simulink model "Accelerator"  (R2022b)
settings: Solver=FixedStepDiscrete  StartTime=0.0  StopTime=10  FixedStep=0.005  RelTol=1e-3  EnableMultiTasking=on
PreLoadFcn:
  | try, model_open; catch, disp('Error occurred while executing model pre-load callback: model_open.m'); disp('Please assure that the MATLAB working directory is set to the model directory before opening.'); end
InitFcn:
  | try, model_open; catch, end
undefined symbols (not defined in the file): GCM, raptor_get_safe_string, raptor_xcp_function
libraries: Raptor_lib x149, simulink x14, Blocks_Library x2, simulink_extras x1
(part 2 of 3)

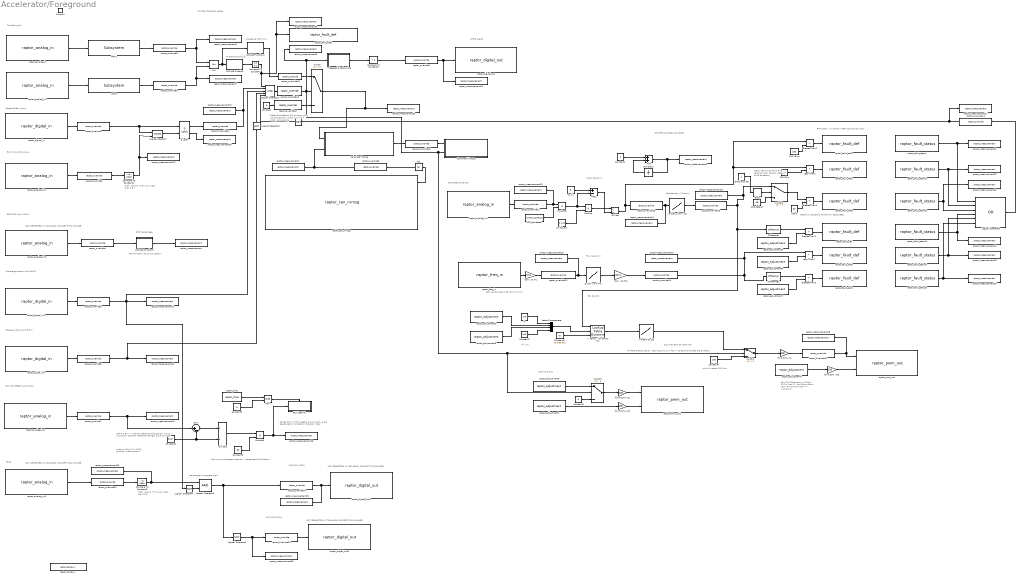
== system Accelerator/Foreground ==
  note: Pre-charge in progress logic
  note: IMD OKHS COIL-
  note: TSMS
  note: NOT REFLECTED IN TOP-LEVEL: COMPETITION CHANGE
  note: Fault function (for some reason)
  note: Throttle enable signal - cooling turns on when Inverter and throttle are enabled
  note: Cooling Pump
  note: Can handle about 4Hz at minimum
  note: Delay temp high fault for 5 seconds upon startup, default to 25 at startup
  note: Resistance in kilo-ohm
  note: Range from +/-50A
      | Negative and positive are dependent on direction of sensor install
  note: Defaults throttle to 0% on error, do not change this unless you know what you're doing
  note: Maximum amperage of sensor, independent of direction
  note: Linearity Error = +/-0.5%
      | Ignored in calculations
  note: Vref = 2.5V --> internal reference
      | Change this value if using an external reference:
      | Range is 0.5 to 2.65V
  note: Averaging POT1 & 2
  note: Throttle Plausibility
  note: Temperature Sensor
  note: Throttle Input
  note: SYSTEM CONTROL CODE
  note: SOC Percentage
  note: High: Above ~2.5V
      | Low: Less than 2.5V
  note: Starter Button Input
  note: Error Input
      | Active Low
  note: BMS SOC Input
      | (0-5V)
  note: Pre-charge Status input
      | (0-5V)
  note: Charge mode input
      | (0-5V)
  note: RTDS Signal
  note: Hold inverted PWM low
  note: Based on Cascadia and Emrax datasheets
  note: Persistent - will remain after VCU power cycle
  note: All in F
  note: assumes 80W @ 100% DC
  note: Flow Sensor In
  note: Fan PWM Frequency is 24KHz
      | 5/(2*pi*tau) --> tau=Larm/Rarm
      | Larm = 0.137mH
      | Rarm = 4.114ohm
  note: Temp Sensor In
  note: Fan Control
  note: DRIVETRAIN COOLING CODE
  note: GLV Hall Effect Input
      | (0-5V)
  note: NOT REFLECTED IN TOP-LEVEL: COMPETITION CHANGE
  note: NOT REFLECTED IN TOP-LEVEL: COMPETITION CHANGE
  note: NOT REFLECTED IN TOP-LEVEL: COMPETITION CHANGE
  note: IMD GLV+ COIL-
  note: High: Above ~2.2V
      | Low: Less than 2.2V
  function : TriggerPort  TriggerType=function-call  VariantControl=(inherit)
  100 C : Constant  Value=80
  100 Ohm : Constant  Value=0.1
  100 kOhm : Constant  Value=100
  25C default : Constant  Value=25
  ADC_corrected : Constant  Value=0.00122100122
  Abs : Abs  SaturateOnIntegerOverflow=off
  Add : Sum
  Add2 : Sum  Inputs=+-
  Calculate Torque : Subsystem
  Command Troque : Subsystem
  Compare To Constant : simulink/Logic and Bit Operations/Compare To Constant  relop=<=  const=0.1  OutDataTypeStr=boolean
  Compare To Constant1 : simulink/Logic and Bit Operations/Compare To Constant  relop=>=  const=2000  OutDataTypeStr=boolean
  Compare To Constant2 : simulink/Logic and Bit Operations/Compare To Constant  relop=>  const=0  OutDataTypeStr=boolean
  Compare To Constant3 : simulink/Logic and Bit Operations/Compare To Constant  relop=>=  const=1800  OutDataTypeStr=boolean
  Constant : Constant  Value=0
  Constant1 : Constant
  Constant2 : Constant  Value=2047
  Constant3 : Constant  Value=50
  Constant4 : Constant  Value=100
  Constant5 : Constant  Value=[0;0;80;80]
  Constant6 : Constant  Value=0
  Constant7 : Constant  Value=149
  Constant8 : Constant  Value=.5
  Conv. to Hz : Gain  Gain=0.01  OutDataTypeStr=uint32  RndMeth=Nearest
  Conv. to Hz1 : Gain  Gain=227.1  OutDataTypeStr=uint32
  D Latch : simulink_extras/Flip Flops/D Latch
  Delay : Delay  DelayLength=1000  InitialCondition=0
  Difference : simulink/Discrete/Difference  ICPrevInput=0.0  OutMin=[]  OutMax=[]  OutDataType=fixdt(1, 16)  OutScaling=2^-10  DoSatur=off
  Difference1 : simulink/Discrete/Difference  ICPrevInput=0.0  OutMin=[]  OutMax=[]  OutDataType=fixdt(1, 16)  OutScaling=2^-10  DoSatur=off
  Divide : Product  Inputs=*/
  Divide1 : Product  Inputs=*/
  Enable switch : Constant
  F : Constant  Value=-18
  GLV Used Ah : Subsystem  TreatAsAtomicUnit=on
  GreaterThan{1..4} (4 alike) : RelationalOperator  Operator=>  OutDataTypeStr=boolean  RndMeth=Simplest  InputSameDT=off
  I: 0-80W O: DC : Lookup_n-D  NumberOfTableDimensions=1  BreakpointsForDimension1=[0;5;10;15;20;25;30;35;40;45;50;55;60;65;70;75;80]  Table=[100;93.75;87.5;81.25;75;68.75;62.5;56.25;50;43.75;37.5;31.25;25;18.75;12.5;6.25;0]  InternalRulePriority=Speed  RndMeth=Simplest
  I: R (kOhm) O: T (C) : Lookup_n-D  NumberOfTableDimensions=1  BreakpointsForDimension1=[0.583;0.6601;0.7487;0.8508;0.9688;1.106;1.265;1.452;1.67;1.928;2.232;2.593;3.025;3.541;4.163;4.914;5.827;6.942;8.311;10;12.1;14.71;17.99;22.13;27.39]  Table=[120;115;110;105;100;95;90;85;80;75;70;65;60;55;50;45;40;35;30;25;20;15;10;5;0]  InternalRulePriority=Speed  RndMeth=Simplest
  I: Temp. () O: Power (W) : simulink/Lookup Tables/Lookup Table Dynamic  LookUpMeth=Interpolation-Use End Values  OutDataType=fixdt('double')  OutScaling=[]  OutputDataTypeScalingMode=Specify via dialog  OutDataTypeStr=double  DoSatur=off
  Less Than1 : RelationalOperator  Operator=<  OutDataTypeStr=boolean  RndMeth=Simplest  InputSameDT=off
  Less Than2 : RelationalOperator  Operator=<  OutDataTypeStr=boolean  RndMeth=Simplest  InputSameDT=off
  Logical Operator : Logic  Operator=NXOR  IconShape=distinctive  AllPortsSameDT=off  OutDataTypeStr=boolean
  Logical Operator1 : Logic  Inputs=5  IconShape=distinctive  AllPortsSameDT=off  OutDataTypeStr=boolean
  Logical Operator{2,4,6..7} (4 alike) : Logic  Operator=NOT  IconShape=distinctive  AllPortsSameDT=off  OutDataTypeStr=boolean
  Logical Operator3 : Logic  Operator=OR  Inputs=6  IconShape=distinctive  AllPortsSameDT=off  OutDataTypeStr=boolean
  Logical Operator5 : Logic  IconShape=distinctive  AllPortsSameDT=off  OutDataTypeStr=boolean
  MATLAB Function : MATLAB Function  TreatAsAtomicUnit=on
  MATLAB Function1 : MATLAB Function  TreatAsAtomicUnit=on
  MATLAB Function2 : MATLAB Function  TreatAsAtomicUnit=on
  Mod : Math  Operator=mod  OutputSignalType=real
  Mux : Mux  Inputs=2
      settings: DisplayOption=signals
  POT1 : Blocks_Library/Subsystem  nam=POT1
  POT2 : Blocks_Library/Subsystem  nam=POT2
  PU (Ohms) : Constant  Value=2.145
  Product : Product
  Product1 : Product
  Product3 : Product
  Q (L/H) vs. F (Hz) : Lookup_n-D  NumberOfTableDimensions=1  BreakpointsForDimension1=[16;32.5;49.3;65.5;82;90.2]  Table=[120;240;360;480;600;720]  ExtrapMethod=Clip  InternalRulePriority=Speed  OutDataTypeStr=double  RndMeth=Simplest
  Sum : Sum  Inputs=|+-
  Switch : Switch  Threshold=1  SaturateOnIntegerOverflow=off  InputSameDT=off
  Switch1 : Switch  Criteria=u2 > Threshold  SaturateOnIntegerOverflow=off  InputSameDT=off
  Switch2 : Switch  Criteria=u2 > Threshold  SaturateOnIntegerOverflow=off  InputSameDT=off
  Switch3 : Switch  Criteria=u2 > Threshold  SaturateOnIntegerOverflow=off  InputSameDT=off
  Triggered Single Pulse : Subsystem  Description=Produce a signal pulse for the RTDS timer circuit  TreatAsAtomicUnit=on  mask(single pulse generation){p_wid=5}
      mask prompts: p_wid "pulse width (number of samples)"
      mask help: This block generate a single pulse whenever a trigger happen. The pulse width must specified as a number of samples. for example if your sampling time is 0.1s and you want 3s pulse , then you should enter 30 as a pulse width.
      mask Display:
      | plot([0],[0])
      | plot([11],[0])
      | plot([5],[0.5])
      | plot([4 5 5 6 6 7],[0 0 0.25 0.25 0 0])
      | plot([5],[-0.3])
      | 
      | port_label('output', 1, 'Pulse')
      | port_label('input', 1, 'Trigger')
  Unit Delay : UnitDelay  SampleTime=-1  HasFrameUpgradeWarning=on
  Vector Concatenate : Concatenate  NumInputs=4
  Vs (V) : Constant  Value=5
  for 0.01% inc{,1..3} (4 alike) : Gain  Gain=100  OutDataTypeStr=Inherit: Inherit via back propagation
  raptor_adjustment1 : Raptor_lib/Data Storage/raptor_adjustment  paramName='Pump_PWM_freq'  nameSource=Parameter  initValue=24000  dataType=uint32  storage=Calibration  calDispType=Number  calEnum={'False', 'True'}  calGain=100  calOffset=0.0  calMax=inf  calMin=-inf  calFormat='-1'  calUnit='Hz'  calHelp=''  calAccess=1  calFunction=raptor_xcp_function(gcb)  calDispHeaders=off  calColHeaders={'Col1' 'Col2' 'Col3'}  calRowHeaders={'Row1' 'Row2' 'Row3'}
      settings: SourceProductName=Raptor
  raptor_adjustment2 : Raptor_lib/Data Storage/raptor_adjustment  paramName='LowerFanPoint'  nameSource=Parameter  initValue=18  dataType=double  storage=Calibration  calDispType=Number  calEnum={'False', 'True'}  calGain=1.0  calOffset=0.0  calMax=inf  calMin=-inf  calFormat='-1'  calUnit='F'  calHelp='Temp at 0W'  calAccess=1  calFunction=raptor_xcp_function(gcb)  calDispHeaders=off  calColHeaders={'Col1' 'Col2' 'Col3'}  calRowHeaders={'Row1' 'Row2' 'Row3'}
      settings: SourceProductName=Raptor
  raptor_adjustment3 : Raptor_lib/Data Storage/raptor_adjustment  paramName='UpperFanPoint'  nameSource=Parameter  initValue=66  dataType=double  storage=Calibration  calDispType=Number  calEnum={'False', 'True'}  calGain=1.0  calOffset=0.0  calMax=inf  calMin=-inf  calFormat='-1'  calUnit='F'  calHelp='Temp at 80W'  calAccess=1  calFunction=raptor_xcp_function(gcb)  calDispHeaders=off  calColHeaders={'Col1' 'Col2' 'Col3'}  calRowHeaders={'Row1' 'Row2' 'Row3'}
      settings: SourceProductName=Raptor
  raptor_adjustment4 : Raptor_lib/Data Storage/raptor_adjustment  paramName='Fan_PWM_freq'  nameSource=Parameter  initValue=24000  dataType=uint32  storage=Calibration  calDispType=Number  calEnum={'False', 'True'}  calGain=100  calOffset=0.0  calMax=inf  calMin=-inf  calFormat='-1'  calUnit='Hz'  calHelp=''  calAccess=1  calFunction=raptor_xcp_function(gcb)  calDispHeaders=off  calColHeaders={'Col1' 'Col2' 'Col3'}  calRowHeaders={'Row1' 'Row2' 'Row3'}
      settings: SourceProductName=Raptor
  raptor_adjustment5 : Raptor_lib/Data Storage/raptor_adjustment  paramName='tempRateFault'  nameSource=Parameter  initValue=10  dataType=double  storage=Calibration  calDispType=Number  calEnum={'False', 'True'}  calGain=1.0  calOffset=0.0  calMax=inf  calMin=-inf  calFormat='-1'  calUnit='degC/sec'  calHelp=''  calAccess=1  calFunction=raptor_xcp_function(gcb)  calDispHeaders=off  calColHeaders={'Col1' 'Col2' 'Col3'}  calRowHeaders={'Row1' 'Row2' 'Row3'}
      settings: SourceProductName=Raptor
  raptor_adjustment6 : Raptor_lib/Data Storage/raptor_adjustment  paramName='lowFlowRateFault'  nameSource=Parameter  initValue=1  dataType=double  storage=Calibration  calDispType=Number  calEnum={'False', 'True'}  calGain=1.0  calOffset=0.0  calMax=inf  calMin=-inf  calFormat='-1'  calUnit='GPM'  calHelp=''  calAccess=1  calFunction=raptor_xcp_function(gcb)  calDispHeaders=off  calColHeaders={'Col1' 'Col2' 'Col3'}  calRowHeaders={'Row1' 'Row2' 'Row3'}
      settings: SourceProductName=Raptor
  raptor_adjustment7 : Raptor_lib/Data Storage/raptor_adjustment  paramName='eradicFlowRateFault'  nameSource=Parameter  initValue=10  dataType=double  storage=Calibration  calDispType=Number  calEnum={'False', 'True'}  calGain=1.0  calOffset=0.0  calMax=inf  calMin=-inf  calFormat='-1'  calUnit='deg/sec'  calHelp=''  calAccess=1  calFunction=raptor_xcp_function(gcb)  calDispHeaders=off  calColHeaders={'Col1' 'Col2' 'Col3'}  calRowHeaders={'Row1' 'Row2' 'Row3'}
      settings: SourceProductName=Raptor
  raptor_adjustment8 : Raptor_lib/Data Storage/raptor_adjustment  paramName='Cooling_pump_PWM_D'  nameSource=Parameter  initValue=0.4  dataType=double  storage=Calibration  calDispType=Number  calEnum={'False', 'True'}  calGain=1.0  calOffset=0.0  calMax=inf  calMin=-inf  calFormat='-1'  calUnit='F'  calHelp='Temp at 80W'  calAccess=1  calFunction=raptor_xcp_function(gcb)  calDispHeaders=off  calColHeaders={'Col1' 'Col2' 'Col3'}  calRowHeaders={'Row1' 'Row2' 'Row3'}
      settings: SourceProductName=Raptor
  raptor_analog_in : Raptor_lib/Input & Output/raptor_analog_in  resourceValues=INPUT2|INPUT3|INPUT4|INPUT5|INPUT6|INPUT7|INPUT8|INPUT9|INPUT10|INPUT11|INPUT12|INPUT13|INPUT14|INPUT15|INPUT16|INPUT17|INPUT18|INPUT19|INPUT20|INPUT21|INPUT22|INPUT23|INPUT24|INPUT25|INPUT26|INPUT27|INPUT28|INPUT29|INPUT30|INPUT31|INPUT32|(None)  resource=INPUT30  rangeValues=0 - 5 V  range=0 - 5 V  filterrateValues=[]  filterrate='RAPTOR MASK DEFAULT'  resolutionValues=[]  resolution=[]  pullUDValues=215k PD  pullUD=215k PD
      settings: SourceProductName=Raptor
  raptor_analog_in1 : Raptor_lib/Input & Output/raptor_analog_in  resourceValues=INPUT2|INPUT3|INPUT4|INPUT5|INPUT6|INPUT7|INPUT8|INPUT9|INPUT10|INPUT11|INPUT12|INPUT13|INPUT14|INPUT15|INPUT16|INPUT17|INPUT18|INPUT19|INPUT20|INPUT21|INPUT22|INPUT23|INPUT24|INPUT25|INPUT26|INPUT27|INPUT28|INPUT29|INPUT30|INPUT31|INPUT32|(None)  resource=INPUT29  rangeValues=0 - 5 V  range=0 - 5 V  filterrateValues=[]  filterrate='RAPTOR MASK DEFAULT'  resolutionValues=[]  resolution=[]  pullUDValues=215k PD  pullUD=215k PD
      settings: SourceProductName=Raptor
  raptor_analog_in2 : Raptor_lib/Input & Output/raptor_analog_in  resourceValues=INPUT2|INPUT3|INPUT4|INPUT5|INPUT6|INPUT7|INPUT8|INPUT9|INPUT10|INPUT11|INPUT12|INPUT13|INPUT14|INPUT15|INPUT16|INPUT17|INPUT18|INPUT19|INPUT20|INPUT21|INPUT22|INPUT23|INPUT24|INPUT25|INPUT26|INPUT27|INPUT28|INPUT29|INPUT30|INPUT31|INPUT32|(None)  resource=INPUT23  rangeValues=0 - 5 V  range=0 - 5 V  filterrateValues=[]  filterrate='RAPTOR MASK DEFAULT'  resolutionValues=[]  resolution=[]  pullUDValues=56.7k PD  pullUD=56.7k PD
      settings: SourceProductName=Raptor
  raptor_analog_in3 : Raptor_lib/Input & Output/raptor_analog_in  resourceValues=INPUT2|INPUT3|INPUT4|INPUT5|INPUT6|INPUT7|INPUT8|INPUT9|INPUT10|INPUT11|INPUT12|INPUT13|INPUT14|INPUT15|INPUT16|INPUT17|INPUT18|INPUT19|INPUT20|INPUT21|INPUT22|INPUT23|INPUT24|INPUT25|INPUT26|INPUT27|INPUT28|INPUT29|INPUT30|INPUT31|INPUT32|(None)  resource=INPUT25  rangeValues=0 - 5 V  range=0 - 5 V  filterrateValues=[]  filterrate='RAPTOR MASK DEFAULT'  resolutionValues=[]  resolution=[]  pullUDValues=2.15k PU  pullUD=2.15k PU
      settings: SourceProductName=Raptor
  raptor_analog_in4 : Raptor_lib/Input & Output/raptor_analog_in  resourceValues=INPUT2|INPUT3|INPUT4|INPUT5|INPUT6|INPUT7|INPUT8|INPUT9|INPUT10|INPUT11|INPUT12|INPUT13|INPUT14|INPUT15|INPUT16|INPUT17|INPUT18|INPUT19|INPUT20|INPUT21|INPUT22|INPUT23|INPUT24|INPUT25|INPUT26|INPUT27|INPUT28|INPUT29|INPUT30|INPUT31|INPUT32|(None)  resource=INPUT21  rangeValues=0 - 5 V  range=0 - 5 V  filterrateValues=[]  filterrate='RAPTOR MASK DEFAULT'  resolutionValues=[]  resolution=[]  pullUDValues=2.15k PU  pullUD=2.15k PU
      settings: SourceProductName=Raptor
  raptor_analog_in5 : Raptor_lib/Input & Output/raptor_analog_in  resourceValues=INPUT2|INPUT3|INPUT4|INPUT5|INPUT6|INPUT7|INPUT8|INPUT9|INPUT10|INPUT11|INPUT12|INPUT13|INPUT14|INPUT15|INPUT16|INPUT17|INPUT18|INPUT19|INPUT20|INPUT21|INPUT22|INPUT23|INPUT24|INPUT25|INPUT26|INPUT27|INPUT28|INPUT29|INPUT30|INPUT31|INPUT32|(None)  resource=INPUT26  rangeValues=0 - 5 V  range=0 - 5 V  filterrateValues=[]  filterrate='RAPTOR MASK DEFAULT'  resolutionValues=[]  resolution=[]  pullUDValues=681k PU  pullUD=681k PU
      settings: SourceProductName=Raptor
  raptor_analog_in6 : Raptor_lib/Input & Output/raptor_analog_in  resourceValues=INPUT2|INPUT3|INPUT4|INPUT5|INPUT6|INPUT7|INPUT8|INPUT9|INPUT10|INPUT11|INPUT12|INPUT13|INPUT14|INPUT15|INPUT16|INPUT17|INPUT18|INPUT19|INPUT20|INPUT21|INPUT22|INPUT23|INPUT24|INPUT25|INPUT26|INPUT27|INPUT28|INPUT29|INPUT30|INPUT31|INPUT32|(None)  resource=INPUT24  rangeValues=0 - 5 V  range=0 - 5 V  filterrateValues=[]  filterrate='RAPTOR MASK DEFAULT'  resolutionValues=[]  resolution=[]  pullUDValues=56.7k PD  pullUD=56.7k PD
      settings: SourceProductName=Raptor
  raptor_can_rxmsg : Raptor_lib/CAN/raptor_can_rxmsg  canDefinition=struct('dbcFile', '20210505 RMS PM and RM CAN DB.dbc','message', 'M165_Motor_Position_Info','comment', '','signals', {{'D1_Motor_Angle_Electrical','D2_Motor_Speed','D3_Electrical_Output_Frequency','D4_Delta_Resolver_Filtered'}},'enabled', [ 1 1 1 1;],'scaled', [ 1 1 1 1;],'canBus', '''CAN1''','messageID', [ 165;],'idMask', [ 536870911;],'payloadMask', [],'payloadValue', [],'period', [ 0;],'mailbox', '''''','queueSize', [ 1;],'label', [ 0;],'ver', [ 2;],'showID', [ 0;],'showRaw', [ 0;],'showRawMsg', [ 0;],'useStartVals', [ 0;],'extendedId', [ 0;],'showAge', [ 0;],'useSimFunc', [ 0;],'sim_func_name', '''''','fill', [ 0;],'editID', [ 0;],'signalOrder', [ 1;],'signalAscDes', [ 1;],'msgLength', [ 8;])  canBus='CAN1'  mailbox=''  payloadMask=[]  payloadValue=[]  idMask=hex2dec('1FFFFFFF')  queueSize=1  showID=0  label=0  fill=0  id=165  showRaw=0  showAge=0  signalOrder=1  signalInfo={{struct('Name', 'D4_Delta_Resolver_Filtered','StartBit', [ 48;],'SignalSize', [ 16;],'ByteOrder', 'LittleEndian','ValueType', 'SIGNED','Class', 'int16','Signed', [ 1;],'Factor', [ 0.1;],'Offset', [ 0;],'Min', [ -3276.8;],'Max', [ 3276.7;],'Units', 'deg','StartVal', [ 0;],'Comment', 'Used in calibration of resolver angle adjustment.','Multiplexed', [ 0;],'Multiplexor', [ 0;],'MultiplexMode_Min', [ 0;],'MultiplexMode_Max', [ 0;]),struct('Name', 'D3_Electrical_Output_Frequency','StartBit', [ 32;],'SignalSize', [ 16;],'ByteOrder', 'LittleEndian','ValueType', 'SIGNED','Class', 'int16','Signed', [ 1;],'Factor', [ 0.1;],'Offset', [ 0;],'Min', [ -3276.8;],'Max', [ 3276.7;],'Units', 'hz','StartVal', [ 0;],'Comment', 'The actual electrical frequency of the inverter','Multiplexed', [ 0;],'Multiplexor', [ 0;],'MultiplexMode_Min', [ 0;],'MultiplexMode_Max', [ 0;]),struct('Name', 'D2_Motor_Speed','StartBit', [ 16;],'SignalSize', [ 16;],'ByteOrder', 'LittleEndian','ValueType', 'SIGNED','Class', 'int16','Signed', [ 1;],'Factor', [ 1;],'Offset', [ 0;],'Min', [ -32768;],'Max', [ 32767;],'Units', 'rpm','StartVal', [ 0;],'Comment', 'The measured speed of the motor','Multiplexed', [ 0;],'Multiplexor', [ 0;],'MultiplexMode_Min', [ 0;],'MultiplexMode_Max', [ 0;]),struct('Name', 'D1_Motor_Angle_Electrical','StartBit', [ 0;],'SignalSize', [ 16;],'ByteOrder', 'LittleEndian','ValueType', 'UNSIGNED','Class', 'uint16','Signed', [ 0;],'Factor', [ 0.1;],'Offset', [ 0;],'Min', [ 0;],'Max', [ 6553.5;],'Units', 'deg','StartVal', [ 0;],'Comment', 'The Electrical Angle of the motor as read by the encoder or resolver','Multiplexed', [ 0;],'Multiplexor', [ 0;],'MultiplexMode_Min', [ 0;],'MultiplexMode_Max', [ 0;])}}  showRawMsg=0  useSimFunc=0  sim_func_name=''  useStartVals=0  extendedId=0
      settings: SourceProductName=Raptor
  raptor_digital_in : Raptor_lib/Input & Output/raptor_digital_in  resourceValues=WAKE_INPUT1|INPUT33|INPUT34|INPUT35|INPUT36|INPUT37|INPUT38|INPUT39|INPUT40|(None)  resource=INPUT37  pullUDValues=1.3k PU  pullUD=1.3k PU  upperThres='RAPTOR MASK DEFAULT'  lowerThres='RAPTOR MASK DEFAULT'
      settings: SourceProductName=Raptor
  raptor_digital_in1 : Raptor_lib/Input & Output/raptor_digital_in  resourceValues=WAKE_INPUT1|INPUT33|INPUT34|INPUT35|INPUT36|INPUT37|INPUT38|INPUT39|INPUT40|(None)  resource=INPUT35  pullUDValues=1.3k PD  pullUD=1.3k PD  upperThres='RAPTOR MASK DEFAULT'  lowerThres='RAPTOR MASK DEFAULT'
      settings: SourceProductName=Raptor
  raptor_digital_in2 : Raptor_lib/Input & Output/raptor_digital_in  resourceValues=WAKE_INPUT1|INPUT33|INPUT34|INPUT35|INPUT36|INPUT37|INPUT38|INPUT39|INPUT40|(None)  resource=INPUT34  pullUDValues=1.3k PD  pullUD=1.3k PD  upperThres='RAPTOR MASK DEFAULT'  lowerThres='RAPTOR MASK DEFAULT'
      settings: SourceProductName=Raptor
  raptor_digital_out : Raptor_lib/Input & Output/raptor_digital_out  resourceValues=OUTPUT1|OUTPUT2|OUTPUT3|OUTPUT4|OUTPUT5|OUTPUT6|OUTPUT7|OUTPUT8|OUTPUT9|OUTPUT10|OUTPUT11|OUTPUT12|OUTPUT21|OUTPUT22|OUTPUT23|OUTPUT24|OUTPUT25|OUTPUT26|OUTPUT27|OUTPUT28|OUTPUT29|OUTPUT30|OUTPUT31|OUTPUT32|OUTPUT33|OUTPUT34|OUTPUT35|OUTPUT36|OUTPUT37|OUTPUT38|OUTPUT39|OUTPUT40|OUTPUT41|OUTPUT42|OUTPUT43|OUTPUT44|OUTPUT45|OUTPUT46|OUTPUT47|OUTPUT48|OUTPUT49|POWER_HOLD|(None)  resource=OUTPUT8  driverTypeValues=Low Side  driverType=Low Side
      settings: SourceProductName=Raptor
  raptor_digital_out1 : Raptor_lib/Input & Output/raptor_digital_out  resourceValues=OUTPUT1|OUTPUT2|OUTPUT3|OUTPUT4|OUTPUT5|OUTPUT6|OUTPUT7|OUTPUT8|OUTPUT9|OUTPUT10|OUTPUT11|OUTPUT12|OUTPUT21|OUTPUT22|OUTPUT23|OUTPUT24|OUTPUT25|OUTPUT26|OUTPUT27|OUTPUT28|OUTPUT29|OUTPUT30|OUTPUT31|OUTPUT32|OUTPUT33|OUTPUT34|OUTPUT35|OUTPUT36|OUTPUT37|OUTPUT38|OUTPUT39|OUTPUT40|OUTPUT41|OUTPUT42|OUTPUT43|OUTPUT44|OUTPUT45|OUTPUT46|OUTPUT47|OUTPUT48|OUTPUT49|POWER_HOLD|(None)  resource=OUTPUT35  driverTypeValues=Low Side  driverType=Low Side
      settings: SourceProductName=Raptor
  raptor_digital_out2 : Raptor_lib/Input & Output/raptor_digital_out  resourceValues=OUTPUT1|OUTPUT2|OUTPUT3|OUTPUT4|OUTPUT5|OUTPUT6|OUTPUT7|OUTPUT8|OUTPUT9|OUTPUT10|OUTPUT11|OUTPUT12|OUTPUT21|OUTPUT22|OUTPUT23|OUTPUT24|OUTPUT25|OUTPUT26|OUTPUT27|OUTPUT28|OUTPUT29|OUTPUT30|OUTPUT31|OUTPUT32|OUTPUT33|OUTPUT34|OUTPUT35|OUTPUT36|OUTPUT37|OUTPUT38|OUTPUT39|OUTPUT40|OUTPUT41|OUTPUT42|OUTPUT43|OUTPUT44|OUTPUT45|OUTPUT46|OUTPUT47|OUTPUT48|OUTPUT49|POWER_HOLD|(None)  resource=OUTPUT38  driverTypeValues=Low Side  driverType=Low Side
      settings: SourceProductName=Raptor
  raptor_fault_def : Raptor_lib/Faults/raptor_fault_def  faultName='eradicTemp'  persist=off  sticky=on  emisRelated=off  singleTrip=off  clearMethod=Standard  xLimit=25  yLimit=50  calEnable=on  addDisable=off  calAccess=1  calFunction='System | FaultManager'
      settings: SourceProductName=Raptor
  raptor_fault_def1 : Raptor_lib/Faults/raptor_fault_def  faultName='tempSenseOC'  persist=off  sticky=off  emisRelated=off  singleTrip=off  clearMethod=Standard  xLimit=25  yLimit=50  calEnable=on  addDisable=off  calAccess=1  calFunction='System | FaultManager'
      settings: SourceProductName=Raptor
  raptor_fault_def2 : Raptor_lib/Faults/raptor_fault_def  faultName='tempSenseSC'  persist=off  sticky=off  emisRelated=off  singleTrip=off  clearMethod=Standard  xLimit=25  yLimit=50  calEnable=on  addDisable=off  calAccess=1  calFunction='System | FaultManager'
      settings: SourceProductName=Raptor
  raptor_fault_def3 : Raptor_lib/Faults/raptor_fault_def  faultName='lowFlowRate'  persist=off  sticky=on  emisRelated=off  singleTrip=off  clearMethod=Standard  xLimit=25  yLimit=50  calEnable=on  addDisable=off  calAccess=1  calFunction='System | FaultManager'
      settings: SourceProductName=Raptor
  raptor_fault_def4 : Raptor_lib/Faults/raptor_fault_def  faultName='eradicFlow'  persist=off  sticky=on  emisRelated=off  singleTrip=off  clearMethod=Standard  xLimit=25  yLimit=50  calEnable=on  addDisable=off  calAccess=1  calFunction='System | FaultManager'
      settings: SourceProductName=Raptor
  raptor_fault_def5 : Raptor_lib/Faults/raptor_fault_def  faultName='tempHigh'  persist=off  sticky=on  emisRelated=off  singleTrip=off  clearMethod=Standard  xLimit=25  yLimit=50  calEnable=on  addDisable=off  calAccess=1  calFunction='System | FaultManager'
      settings: SourceProductName=Raptor
  raptor_fault_def6 : Raptor_lib/Faults/raptor_fault_def  faultName='Throttle_plausibility'  persist=off  sticky=on  emisRelated=off  singleTrip=off  clearMethod=Standard  xLimit=25  yLimit=50  calEnable=on  addDisable=off  calAccess=1  calFunction='System | FaultManager'
      settings: SourceProductName=Raptor
  raptor_fault_status : Raptor_lib/Faults/raptor_fault_status  faultSource=Parameter  faultName='tempSenseOC'  notOccurred=off  suspected=off  active=on  occurred=off  failedThisDC=off  testCmpltThisDC=off  failing=off  pending=on  confirmed=on  mil=on  permanent=off  ready=on  prevConfirmed=off  failedSinceClear=off  failedLastDC=off  prevMil=off
      settings: SourceProductName=Raptor
  raptor_fault_status1 : Raptor_lib/Faults/raptor_fault_status  faultSource=Parameter  faultName='tempSenseSC'  notOccurred=off  suspected=off  active=on  occurred=off  failedThisDC=off  testCmpltThisDC=off  failing=off  pending=on  confirmed=on  mil=on  permanent=off  ready=on  prevConfirmed=off  failedSinceClear=off  failedLastDC=off  prevMil=off
      settings: SourceProductName=Raptor
  raptor_fault_status2 : Raptor_lib/Faults/raptor_fault_status  faultSource=Parameter  faultName='tempHigh'  notOccurred=off  suspected=off  active=on  occurred=off  failedThisDC=off  testCmpltThisDC=off  failing=off  pending=on  confirmed=on  mil=on  permanent=off  ready=on  prevConfirmed=off  failedSinceClear=off  failedLastDC=off  prevMil=off
      settings: SourceProductName=Raptor
  raptor_fault_status3 : Raptor_lib/Faults/raptor_fault_status  faultSource=Parameter  faultName='eradicTemp'  notOccurred=off  suspected=off  active=on  occurred=off  failedThisDC=off  testCmpltThisDC=off  failing=off  pending=on  confirmed=on  mil=on  permanent=off  ready=on  prevConfirmed=off  failedSinceClear=off  failedLastDC=off  prevMil=off
      settings: SourceProductName=Raptor
  raptor_fault_status4 : Raptor_lib/Faults/raptor_fault_status  faultSource=Parameter  faultName='lowFlowRate'  notOccurred=off  suspected=off  active=on  occurred=off  failedThisDC=off  testCmpltThisDC=off  failing=off  pending=on  confirmed=on  mil=on  permanent=off  ready=on  prevConfirmed=off  failedSinceClear=off  failedLastDC=off  prevMil=off
      settings: SourceProductName=Raptor
  raptor_fault_status5 : Raptor_lib/Faults/raptor_fault_status  faultSource=Parameter  faultName='eradicFlow'  notOccurred=off  suspected=off  active=on  occurred=off  failedThisDC=off  testCmpltThisDC=off  failing=off  pending=on  confirmed=on  mil=on  permanent=off  ready=on  prevConfirmed=off  failedSinceClear=off  failedLastDC=off  prevMil=off
      settings: SourceProductName=Raptor
  raptor_freq_in : Raptor_lib/Input & Output/raptor_freq_in  minFreq=1  resourceValues=INPUT41|INPUT42|INPUT43|INPUT44|INPUT45|(None)  resource=INPUT43  pullUDValues=[]  pullUD=[]  interfaceValues=[]  interface=[]  hasDuty=off  hasEdgeCount='RAPTOR MASK DEFAULT'
      settings: SourceProductName=Raptor
  raptor_measurement : Raptor_lib/Data Storage/raptor_measurement  paramName='BMS_SOC_percent'  nameSource=Parameter  calDispType=Number  calEnum={'False', 'True'}  calGain=1.0  calOffset=0.0  calMax=inf  calMin=-inf  calFormat='-1'  calUnit=''  calHelp=''  calAccess=1  calFunction=raptor_xcp_function(gcb)  calVisible=on
      settings: SourceProductName=Raptor
  raptor_measurement1 : Raptor_lib/Data Storage/raptor_measurement  paramName='Precharge_status'  nameSource=Parameter  calDispType=Number  calEnum={'False', 'True'}  calGain=1.0  calOffset=0.0  calMax=inf  calMin=-inf  calFormat='-1'  calUnit=''  calHelp=''  calAccess=1  calFunction=raptor_xcp_function(gcb)  calVisible=on
      settings: SourceProductName=Raptor
  raptor_measurement10 : Raptor_lib/Data Storage/raptor_measurement  paramName='Starter_button'  nameSource=Parameter  calDispType=Number  calEnum={'False', 'True'}  calGain=1.0  calOffset=0.0  calMax=inf  calMin=-inf  calFormat='-1'  calUnit=''  calHelp=''  calAccess=1  calFunction=raptor_xcp_function(gcb)  calVisible=on
      settings: SourceProductName=Raptor
  raptor_measurement11 : Raptor_lib/Data Storage/raptor_measurement  paramName='Safety_loop_error_logic'  nameSource=Parameter  calDispType=Number  calEnum={'False', 'True'}  calGain=1.0  calOffset=0.0  calMax=inf  calMin=-inf  calFormat='-1'  calUnit=''  calHelp=''  calAccess=1  calFunction=raptor_xcp_function(gcb)  calVisible=on
      settings: SourceProductName=Raptor
  raptor_measurement12 : Raptor_lib/Data Storage/raptor_measurement  paramName='RTDS'  nameSource=Parameter  calDispType=Number  calEnum={'False', 'True'}  calGain=1.0  calOffset=0.0  calMax=inf  calMin=-inf  calFormat='-1'  calUnit=''  calHelp=''  calAccess=1  calFunction=raptor_xcp_function(gcb)  calVisible=on
      settings: SourceProductName=Raptor
  raptor_measurement13 : Raptor_lib/Data Storage/raptor_measurement  paramName='Temp_adc_raw'  nameSource=Parameter  calDispType=Number  calEnum={'False', 'True'}  calGain=1.0  calOffset=0.0  calMax=inf  calMin=-inf  calFormat='-1'  calUnit=''  calHelp=''  calAccess=1  calFunction=raptor_xcp_function(gcb)  calVisible=on
      settings: SourceProductName=Raptor
  raptor_measurement14 : Raptor_lib/Data Storage/raptor_measurement  paramName='Temp_resistance'  nameSource=Parameter  calDispType=Number  calEnum={'False', 'True'}  calGain=1.0  calOffset=0.0  calMax=inf  calMin=-inf  calFormat='-1'  calUnit=''  calHelp=''  calAccess=1  calFunction=raptor_xcp_function(gcb)  calVisible=on
      settings: SourceProductName=Raptor
  raptor_measurement15 : Raptor_lib/Data Storage/raptor_measurement  paramName='GLV_hall_adc'  nameSource=Parameter  calDispType=Number  calEnum={'False', 'True'}  calGain=1.0  calOffset=0.0  calMax=inf  calMin=-inf  calFormat='-1'  calUnit=''  calHelp=''  calAccess=1  calFunction=raptor_xcp_function(gcb)  calVisible=on
      settings: SourceProductName=Raptor
  raptor_measurement16 : Raptor_lib/Data Storage/raptor_measurement  paramName='GLV_hall_amp'  nameSource=Parameter  calDispType=Number  calEnum={'False', 'True'}  calGain=1.0  calOffset=0.0  calMax=inf  calMin=-inf  calFormat='-1'  calUnit=''  calHelp=''  calAccess=1  calFunction=raptor_xcp_function(gcb)  calVisible=on
      settings: SourceProductName=Raptor
  raptor_measurement17 : Raptor_lib/Data Storage/raptor_measurement  paramName='Cooling_fault_any'  nameSource=Parameter  calDispType=Number  calEnum={'False', 'True'}  calGain=1.0  calOffset=0.0  calMax=inf  calMin=-inf  calFormat='-1'  calUnit=''  calHelp=''  calAccess=1  calFunction=raptor_xcp_function(gcb)  calVisible=on
      settings: SourceProductName=Raptor
  raptor_measurement18 : Raptor_lib/Data Storage/raptor_measurement  paramName='Flow_rate_freq_corrected'  nameSource=Parameter  calDispType=Number  calEnum={'False', 'True'}  calGain=1.0  calOffset=0.0  calMax=inf  calMin=-inf  calFormat='-1'  calUnit=''  calHelp=''  calAccess=1  calFunction=raptor_xcp_function(gcb)  calVisible=on
      settings: SourceProductName=Raptor
  raptor_measurement19 : Raptor_lib/Data Storage/raptor_measurement  paramName='Flow_rate_gpm'  nameSource=Parameter  calDispType=Number  calEnum={'False', 'True'}  calGain=1.0  calOffset=0.0  calMax=inf  calMin=-inf  calFormat='-1'  calUnit=''  calHelp=''  calAccess=1  calFunction=raptor_xcp_function(gcb)  calVisible=on
      settings: SourceProductName=Raptor
  raptor_measurement2 : Raptor_lib/Data Storage/raptor_measurement  paramName='Charge_mode'  nameSource=Parameter  calDispType=Number  calEnum={'False', 'True'}  calGain=1.0  calOffset=0.0  calMax=inf  calMin=-inf  calFormat='-1'  calUnit=''  calHelp=''  calAccess=1  calFunction=raptor_xcp_function(gcb)  calVisible=on
      settings: SourceProductName=Raptor
  raptor_measurement20 : Raptor_lib/Data Storage/raptor_measurement  paramName='Starter_button_latch_q_naught'  nameSource=Parameter  calDispType=Number  calEnum={'False', 'True'}  calGain=1.0  calOffset=0.0  calMax=inf  calMin=-inf  calFormat='-1'  calUnit=''  calHelp=''  calAccess=1  calFunction=raptor_xcp_function(gcb)  calVisible=on
      settings: SourceProductName=Raptor
  raptor_measurement21 : Raptor_lib/Data Storage/raptor_measurement  paramName='fault_tempSenseOC'  nameSource=Parameter  calDispType=Number  calEnum={'False', 'True'}  calGain=1.0  calOffset=0.0  calMax=inf  calMin=-inf  calFormat='-1'  calUnit=''  calHelp=''  calAccess=1  calFunction=raptor_xcp_function(gcb)  calVisible=on
      settings: SourceProductName=Raptor
  raptor_measurement22 : Raptor_lib/Data Storage/raptor_measurement  paramName='fault_tempSenseSC'  nameSource=Parameter  calDispType=Number  calEnum={'False', 'True'}  calGain=1.0  calOffset=0.0  calMax=inf  calMin=-inf  calFormat='-1'  calUnit=''  calHelp=''  calAccess=1  calFunction=raptor_xcp_function(gcb)  calVisible=on
      settings: SourceProductName=Raptor
  raptor_measurement23 : Raptor_lib/Data Storage/raptor_measurement  paramName='fault_tempSenseHigh'  nameSource=Parameter  calDispType=Number  calEnum={'False', 'True'}  calGain=1.0  calOffset=0.0  calMax=inf  calMin=-inf  calFormat='-1'  calUnit=''  calHelp=''  calAccess=1  calFunction=raptor_xcp_function(gcb)  calVisible=on
      settings: SourceProductName=Raptor
  raptor_measurement24 : Raptor_lib/Data Storage/raptor_measurement  paramName='fault_eradic_temp'  nameSource=Parameter  calDispType=Number  calEnum={'False', 'True'}  calGain=1.0  calOffset=0.0  calMax=inf  calMin=-inf  calFormat='-1'  calUnit=''  calHelp=''  calAccess=1  calFunction=raptor_xcp_function(gcb)  calVisible=on
      settings: SourceProductName=Raptor
  raptor_measurement25 : Raptor_lib/Data Storage/raptor_measurement  paramName='fault_lowFlowRate'  nameSource=Parameter  calDispType=Number  calEnum={'False', 'True'}  calGain=1.0  calOffset=0.0  calMax=inf  calMin=-inf  calFormat='-1'  calUnit=''  calHelp=''  calAccess=1  calFunction=raptor_xcp_function(gcb)  calVisible=on
      settings: SourceProductName=Raptor
  raptor_measurement26 : Raptor_lib/Data Storage/raptor_measurement  paramName='fault_eradicFlowRate'  nameSource=Parameter  calDispType=Number  calEnum={'False', 'True'}  calGain=1.0  calOffset=0.0  calMax=inf  calMin=-inf  calFormat='-1'  calUnit=''  calHelp=''  calAccess=1  calFunction=raptor_xcp_function(gcb)  calVisible=on
      settings: SourceProductName=Raptor
  raptor_measurement27 : Raptor_lib/Data Storage/raptor_measurement  paramName='Temp_actual_celsius'  nameSource=Parameter  calDispType=Number  calEnum={'False', 'True'}  calGain=1.0  calOffset=0.0  calMax=inf  calMin=-inf  calFormat='-1'  calUnit=''  calHelp=''  calAccess=4  calFunction=raptor_xcp_function(gcb)  calVisible=on
      settings: SourceProductName=Raptor
  raptor_measurement28 : Raptor_lib/Data Storage/raptor_measurement  paramName='Fan_PWM_D'  nameSource=Parameter  calDispType=Number  calEnum={'False', 'True'}  calGain=1.0  calOffset=0.0  calMax=inf  calMin=-inf  calFormat='-1'  calUnit=''  calHelp=''  calAccess=1  calFunction=raptor_xcp_function(gcb)  calVisible=on
      settings: SourceProductName=Raptor
  raptor_measurement29 : Raptor_lib/Data Storage/raptor_measurement  paramName='TSMS_logic_probe'  nameSource=Parameter  calDispType=Number  calEnum={'False', 'True'}  calGain=1.0  calOffset=0.0  calMax=inf  calMin=-inf  calFormat='-1'  calUnit=''  calHelp=''  calAccess=1  calFunction=raptor_xcp_function(gcb)  calVisible=on
      settings: SourceProductName=Raptor
  raptor_measurement3 : Raptor_lib/Data Storage/raptor_measurement  paramName='Counter'  nameSource=Parameter  calDispType=Number  calEnum={'False', 'True'}  calGain=1.0  calOffset=0.0  calMax=inf  calMin=-inf  calFormat='-1'  calUnit=''  calHelp=''  calAccess=4  calFunction=raptor_xcp_function(gcb)  calVisible=on
      settings: SourceProductName=Raptor
  raptor_measurement30 : Raptor_lib/Data Storage/raptor_measurement  paramName='IMD_OkHs_probe'  nameSource=Parameter  calDispType=Number  calEnum={'False', 'True'}  calGain=1.0  calOffset=0.0  calMax=inf  calMin=-inf  calFormat='-1'  calUnit=''  calHelp=''  calAccess=1  calFunction=raptor_xcp_function(gcb)  calVisible=on
      settings: SourceProductName=Raptor
  raptor_measurement31 : Raptor_lib/Data Storage/raptor_measurement  paramName='IMD_GLV_probe'  nameSource=Parameter  calDispType=Number  calEnum={'False', 'True'}  calGain=1.0  calOffset=0.0  calMax=inf  calMin=-inf  calFormat='-1'  calUnit=''  calHelp=''  calAccess=1  calFunction=raptor_xcp_function(gcb)  calVisible=on
      settings: SourceProductName=Raptor
  raptor_measurement4 : Raptor_lib/Data Storage/raptor_measurement  paramName='RPM_val'  nameSource=Parameter  calDispType=Number  calEnum={'False', 'True'}  calGain=1.0  calOffset=0.0  calMax=inf  calMin=-inf  calFormat='-1'  calUnit=''  calHelp=''  calAccess=1  calFunction=raptor_xcp_function(gcb)  calVisible=on
      settings: SourceProductName=Raptor
  raptor_measurement5 : Raptor_lib/Data Storage/raptor_measurement  paramName='TP_val'  nameSource=Parameter  calDispType=Number  calEnum={'False', 'True'}  calGain=1.0  calOffset=0.0  calMax=inf  calMin=-inf  calFormat='-1'  calUnit=''  calHelp=''  calAccess=1  calFunction=raptor_xcp_function(gcb)  calVisible=on
      settings: SourceProductName=Raptor
  raptor_measurement6 : Raptor_lib/Data Storage/raptor_measurement  paramName='APP1'  nameSource=Parameter  calDispType=Number  calEnum={'False', 'True'}  calGain=1.0  calOffset=0.0  calMax=inf  calMin=-inf  calFormat='-1'  calUnit=''  calHelp=''  calAccess=1  calFunction=raptor_xcp_function(gcb)  calVisible=on
      settings: SourceProductName=Raptor
  raptor_measurement7 : Raptor_lib/Data Storage/raptor_measurement  paramName='APP2'  nameSource=Parameter  calDispType=Number  calEnum={'False', 'True'}  calGain=1.0  calOffset=0.0  calMax=inf  calMin=-inf  calFormat='-1'  calUnit=''  calHelp=''  calAccess=1  calFunction=raptor_xcp_function(gcb)  calVisible=on
      settings: SourceProductName=Raptor
  raptor_measurement8 : Raptor_lib/Data Storage/raptor_measurement  paramName='Throttle_plausibility_probe'  nameSource=Parameter  calDispType=Number  calEnum={'False', 'True'}  calGain=1.0  calOffset=0.0  calMax=inf  calMin=-inf  calFormat='-1'  calUnit=''  calHelp=''  calAccess=1  calFunction=raptor_xcp_function(gcb)  calVisible=on
      settings: SourceProductName=Raptor
  raptor_measurement9 : Raptor_lib/Data Storage/raptor_measurement  paramName='Drive_enable'  nameSource=Parameter  calDispType=Number  calEnum={'False', 'True'}  calGain=1.0  calOffset=0.0  calMax=inf  calMin=-inf  calFormat='-1'  calUnit=''  calHelp=''  calAccess=1  calFunction=raptor_xcp_function(gcb)  calVisible=on
      settings: SourceProductName=Raptor
  raptor_override : Raptor_lib/Data Storage/raptor_override  paramName='Starter_button_raw_override'  nameSource=Parameter  measurement=None  calDispType=Number  calEnum={'False', 'True'}  calGain=1.0  calOffset=0.0  calMax=inf  calMin=-inf  calFormat='-1'  calUnit=''  calHelp=''  calAccess=1  calFunction="[raptor_xcp_function(gcb) '|'  'Override']"
      settings: SourceProductName=Raptor
  raptor_override1 : Raptor_lib/Data Storage/raptor_override  paramName='Safety_loop_error_raw_override'  nameSource=Parameter  measurement=None  calDispType=Number  calEnum={'False', 'True'}  calGain=1.0  calOffset=0.0  calMax=inf  calMin=-inf  calFormat='-1'  calUnit=''  calHelp=''  calAccess=1  calFunction="[raptor_xcp_function(gcb) '|'  'Override']"
      settings: SourceProductName=Raptor
  raptor_override10 : Raptor_lib/Data Storage/raptor_override  paramName='Drive_enable_override'  nameSource=Parameter  measurement=None  calDispType=Number  calEnum={'False', 'True'}  calGain=1.0  calOffset=0.0  calMax=inf  calMin=-inf  calFormat='-1'  calUnit=''  calHelp=''  calAccess=1  calFunction="[raptor_xcp_function(gcb) '|'  'Override']"
      settings: SourceProductName=Raptor
  raptor_override11 : Raptor_lib/Data Storage/raptor_override  paramName='Starter_button_override'  nameSource=Parameter  measurement=None  calDispType=Number  calEnum={'False', 'True'}  calGain=1.0  calOffset=0.0  calMax=inf  calMin=-inf  calFormat='-1'  calUnit=''  calHelp=''  calAccess=1  calFunction="[raptor_xcp_function(gcb) '|'  'Override']"
      settings: SourceProductName=Raptor
  raptor_override12 : Raptor_lib/Data Storage/raptor_override  paramName='Temp_adc_raw_override'  nameSource=Parameter  measurement=None  calDispType=Number  calEnum={'False', 'True'}  calGain=1.0  calOffset=0.0  calMax=inf  calMin=-inf  calFormat='-1'  calUnit=''  calHelp=''  calAccess=1  calFunction="[raptor_xcp_function(gcb) '|'  'Override']"
      settings: SourceProductName=Raptor
  raptor_override13 : Raptor_lib/Data Storage/raptor_override  paramName='Temp_resistance_override'  nameSource=Parameter  measurement=None  calDispType=Number  calEnum={'False', 'True'}  calGain=1.0  calOffset=0.0  calMax=inf  calMin=-inf  calFormat='-1'  calUnit=''  calHelp=''  calAccess=1  calFunction="[raptor_xcp_function(gcb) '|'  'Override']"
      settings: SourceProductName=Raptor
  raptor_override14 : Raptor_lib/Data Storage/raptor_override  paramName='Cooling_fault_any_override'  nameSource=Parameter  measurement=None  calDispType=Number  calEnum={'False', 'True'}  calGain=1.0  calOffset=0.0  calMax=inf  calMin=-inf  calFormat='-1'  calUnit=''  calHelp=''  calAccess=1  calFunction="[raptor_xcp_function(gcb) '|'  'Override']"
      settings: SourceProductName=Raptor
  raptor_override15 : Raptor_lib/Data Storage/raptor_override  paramName='APP_override'  nameSource=Parameter  measurement=None  calDispType=Number  calEnum={'False', 'True'}  calGain=1.0  calOffset=0.0  calMax=inf  calMin=-inf  calFormat='-1'  calUnit=''  calHelp=''  calAccess=1  calFunction="[raptor_xcp_function(gcb) '|'  'Override']"
      settings: SourceProductName=Raptor
  raptor_override16 : Raptor_lib/Data Storage/raptor_override  paramName='Torque_map_val_override'  nameSource=Parameter  measurement=None  calDispType=Number  calEnum={'False', 'True'}  calGain=1.0  calOffset=0.0  calMax=inf  calMin=-inf  calFormat='-1'  calUnit=''  calHelp=''  calAccess=1  calFunction="[raptor_xcp_function(gcb) '|'  'Override']"
      settings: SourceProductName=Raptor
  raptor_override17 : Raptor_lib/Data Storage/raptor_override  paramName='APP_default_err_override'  nameSource=Parameter  measurement=None  calDispType=Number  calEnum={'False', 'True'}  calGain=1.0  calOffset=0.0  calMax=inf  calMin=-inf  calFormat='-1'  calUnit=''  calHelp=''  calAccess=1  calFunction="[raptor_xcp_function(gcb) '|'  'Override']"
      settings: SourceProductName=Raptor
  raptor_override18 : Raptor_lib/Data Storage/raptor_override  paramName='Temp_actual_celsius_override'  nameSource=Parameter  measurement=None  calDispType=Number  calEnum={'False', 'True'}  calGain=1.0  calOffset=0.0  calMax=inf  calMin=-inf  calFormat='-1'  calUnit=''  calHelp=''  calAccess=1  calFunction="[raptor_xcp_function(gcb) '|'  'Override']"
      settings: SourceProductName=Raptor
  raptor_override19 : Raptor_lib/Data Storage/raptor_override  paramName='Flow_rate_gpm_override'  nameSource=Parameter  measurement=None  calDispType=Number  calEnum={'False', 'True'}  calGain=1.0  calOffset=0.0  calMax=inf  calMin=-inf  calFormat='-1'  calUnit=''  calHelp=''  calAccess=1  calFunction="[raptor_xcp_function(gcb) '|'  'Override']"
      settings: SourceProductName=Raptor
  raptor_override2 : Raptor_lib/Data Storage/raptor_override  paramName='RTDS_override'  nameSource=Parameter  measurement=None  calDispType=Number  calEnum={'False', 'True'}  calGain=1.0  calOffset=0.0  calMax=inf  calMin=-inf  calFormat='-1'  calUnit=''  calHelp=''  calAccess=1  calFunction="[raptor_xcp_function(gcb) '|'  'Override']"
      settings: SourceProductName=Raptor
  raptor_override20 : Raptor_lib/Data Storage/raptor_override  paramName='Flowrate_hz_corrected_override'  nameSource=Parameter  measurement=None  calDispType=Number  calEnum={'False', 'True'}  calGain=1.0  calOffset=0.0  calMax=inf  calMin=-inf  calFormat='-1'  calUnit=''  calHelp=''  calAccess=1  calFunction="[raptor_xcp_function(gcb) '|'  'Override']"
      settings: SourceProductName=Raptor
  raptor_override21 : Raptor_lib/Data Storage/raptor_override  paramName='Fan_PWM_D_override'  nameSource=Parameter  measurement=None  calDispType=Number  calEnum={'False', 'True'}  calGain=1.0  calOffset=0.0  calMax=inf  calMin=-inf  calFormat='-1'  calUnit=''  calHelp=''  calAccess=1  calFunction="[raptor_xcp_function(gcb) '|'  'Override']"
      settings: SourceProductName=Raptor
  raptor_override22 : Raptor_lib/Data Storage/raptor_override  paramName='TSMS_ADC_override'  nameSource=Parameter  measurement=None  calDispType=Number  calEnum={'False', 'True'}  calGain=1.0  calOffset=0.0  calMax=inf  calMin=-inf  calFormat='-1'  calUnit=''  calHelp=''  calAccess=1  calFunction="[raptor_xcp_function(gcb) '|'  'Override']"
      settings: SourceProductName=Raptor
  raptor_override23 : Raptor_lib/Data Storage/raptor_override  paramName='IMD_OkHs_override'  nameSource=Parameter  measurement=None  calDispType=Number  calEnum={'False', 'True'}  calGain=1.0  calOffset=0.0  calMax=inf  calMin=-inf  calFormat='-1'  calUnit=''  calHelp=''  calAccess=1  calFunction="[raptor_xcp_function(gcb) '|'  'Override']"
      settings: SourceProductName=Raptor
  raptor_override24 : Raptor_lib/Data Storage/raptor_override  paramName='IMD_GLV_override'  nameSource=Parameter  measurement=None  calDispType=Number  calEnum={'False', 'True'}  calGain=1.0  calOffset=0.0  calMax=inf  calMin=-inf  calFormat='-1'  calUnit=''  calHelp=''  calAccess=1  calFunction="[raptor_xcp_function(gcb) '|'  'Override']"
      settings: SourceProductName=Raptor
  raptor_override3 : Raptor_lib/Data Storage/raptor_override  paramName='RPM_override'  nameSource=Parameter  measurement=None  calDispType=Number  calEnum={'False', 'True'}  calGain=1.0  calOffset=0.0  calMax=inf  calMin=-inf  calFormat='-1'  calUnit=''  calHelp=''  calAccess=1  calFunction="[raptor_xcp_function(gcb) '|'  'Override']"
      settings: SourceProductName=Raptor
  raptor_override4 : Raptor_lib/Data Storage/raptor_override  paramName='BMS_SOC_raw_override'  nameSource=Parameter  measurement=None  calDispType=Number  calEnum={'False', 'True'}  calGain=1.0  calOffset=0.0  calMax=inf  calMin=-inf  calFormat='-1'  calUnit=''  calHelp=''  calAccess=1  calFunction="[raptor_xcp_function(gcb) '|'  'Override']"
      settings: SourceProductName=Raptor
  raptor_override5 : Raptor_lib/Data Storage/raptor_override  paramName='Precharge_raw_override'  nameSource=Parameter  measurement=None  calDispType=Number  calEnum={'False', 'True'}  calGain=1.0  calOffset=0.0  calMax=inf  calMin=-inf  calFormat='-1'  calUnit=''  calHelp=''  calAccess=1  calFunction="[raptor_xcp_function(gcb) '|'  'Override']"
      settings: SourceProductName=Raptor
  raptor_override6 : Raptor_lib/Data Storage/raptor_override  paramName='Charge_mode_raw_override'  nameSource=Parameter  measurement=None  calDispType=Number  calEnum={'False', 'True'}  calGain=1.0  calOffset=0.0  calMax=inf  calMin=-inf  calFormat='-1'  calUnit=''  calHelp=''  calAccess=1  calFunction="[raptor_xcp_function(gcb) '|'  'Override']"
      settings: SourceProductName=Raptor
  raptor_override7 : Raptor_lib/Data Storage/raptor_override  paramName='GLV_hall_out_raw_override'  nameSource=Parameter  measurement=None  calDispType=Number  calEnum={'False', 'True'}  calGain=1.0  calOffset=0.0  calMax=inf  calMin=-inf  calFormat='-1'  calUnit=''  calHelp=''  calAccess=1  calFunction="[raptor_xcp_function(gcb) '|'  'Override']"
      settings: SourceProductName=Raptor
  raptor_override8 : Raptor_lib/Data Storage/raptor_override  paramName='APP1_override'  nameSource=Parameter  measurement=None  calDispType=Number  calEnum={'False', 'True'}  calGain=1.0  calOffset=0.0  calMax=inf  calMin=-inf  calFormat='-1'  calUnit=''  calHelp=''  calAccess=1  calFunction="[raptor_xcp_function(gcb) '|'  'Override']"
      settings: SourceProductName=Raptor
  raptor_override9 : Raptor_lib/Data Storage/raptor_override  paramName='APP2_override'  nameSource=Parameter  measurement=None  calDispType=Number  calEnum={'False', 'True'}  calGain=1.0  calOffset=0.0  calMax=inf  calMin=-inf  calFormat='-1'  calUnit=''  calHelp=''  calAccess=1  calFunction="[raptor_xcp_function(gcb) '|'  'Override']"
      settings: SourceProductName=Raptor
  raptor_pwm_out : Raptor_lib/Input & Output/raptor_pwm_out  showEnable=0  resourceValues=OUTPUT1|OUTPUT2|OUTPUT3|OUTPUT4|OUTPUT5|OUTPUT6|OUTPUT7|OUTPUT8|OUTPUT9|OUTPUT10|OUTPUT11|OUTPUT12|(None)  resource=OUTPUT11  driverTypeValues=Low Side  driverType=Low Side
      settings: SourceProductName=Raptor
  raptor_pwm_out1 : Raptor_lib/Input & Output/raptor_pwm_out  showEnable=0  resourceValues=OUTPUT1|OUTPUT2|OUTPUT3|OUTPUT4|OUTPUT5|OUTPUT6|OUTPUT7|OUTPUT8|OUTPUT9|OUTPUT10|OUTPUT11|OUTPUT12|(None)  resource=OUTPUT7  driverTypeValues=Low Side  driverType=Low Side
      settings: SourceProductName=Raptor
  raptor_store_nv : Raptor_lib/Data Storage/raptor_store_nv  null=0
      settings: SourceProductName=Raptor
  raptor_time : Raptor_lib/Triggers/raptor_time  unit=seconds
      settings: SourceProductName=Raptor
  wires:
  Logical Operator/1 -> D Latch/2
  Mux/1 -> MATLAB Function1/1(u), MATLAB Function/1(u)
  POT1/1 -> raptor_override8/1  "u(1)"
  POT2/1 -> raptor_override9/1  "u(2)"
  MATLAB Function/1(y) -> Compare To Constant/1
  Logical Operator1/1 -> raptor_override10/1
  Compare To Constant/1 -> raptor_measurement8/1, raptor_fault_def6/1, Logical Operator1/1
  D Latch/1 -> raptor_override11/1
  Constant/1 -> raptor_override17/1
  MATLAB Function1/1(y) -> raptor_override15/1
  raptor_can_rxmsg/1 -> Abs/1
  D Latch/2 -> raptor_measurement20/1
  raptor_override/1 -> D Latch/1, Logical Operator/1
  raptor_digital_in/1 -> raptor_override/1
  raptor_analog_in2/1 -> raptor_override1/1
  raptor_override1/1 -> Compare To Constant1/1
  raptor_analog_in3/1 -> raptor_override4/1
  raptor_override4/1 -> MATLAB Function2/1(u)
  MATLAB Function2/1(y) -> raptor_measurement/1
  raptor_digital_in1/1 -> raptor_override5/1
  raptor_override5/1 -> Logical Operator4/1, raptor_measurement1/1, Logical Operator1/3
  raptor_digital_in2/1 -> raptor_override6/1
  Logical Operator2/1 -> Logical Operator1/4
  raptor_override6/1 -> raptor_measurement2/1, Logical Operator2/1
  Triggered Single Pulse/1(Pulse) -> Compare To Constant2/1
  raptor_analog_in4/1 -> raptor_override12/1
  Product3/1 -> Add2/2, Product/1
  ADC_corrected/1 -> Product3/2
  100 kOhm/1 -> GreaterThan2/2
  Vector Concatenate/1 -> I: Temp. () O: Power (W)/2
  I: Temp. () O: Power (W)/1 -> I: 0-80W O: DC/1
  Divide/1 -> Less Than1/1, GreaterThan2/1, raptor_override13/1
  Constant5/1 -> I: Temp. () O: Power (W)/3
  100 C/1 -> GreaterThan4/2
  GreaterThan4/1 -> raptor_fault_def5/1
  Difference1/1 -> GreaterThan3/1
  raptor_adjustment7/1 -> GreaterThan3/2
  raptor_adjustment6/1 -> Less Than2/2
  GreaterThan3/1 -> raptor_fault_def4/1
  raptor_adjustment3/1 -> Vector Concatenate/3
  PU (Ohms)/1 -> Product/2
  raptor_freq_in/1 -> Conv. to Hz/1
  Less Than2/1 -> raptor_fault_def3/1
  Product/1 -> Divide/1
  I: R (kOhm) O: T (C)/1 -> raptor_override18/1
  F/1 -> Vector Concatenate/1
  Switch1/1 -> for 0.01% inc/1
  Less Than1/1 -> raptor_fault_def2/1
  100 Ohm/1 -> Less Than1/2
  Vs (V)/1 -> Add2/1
  raptor_adjustment2/1 -> Vector Concatenate/2
  Unit Delay/1 -> Add/2
  Add/1 -> raptor_measurement3/1, Unit Delay/1
  raptor_adjustment4/1 -> for 0.01% inc3/1
  GreaterThan2/1 -> raptor_fault_def1/1
  Difference/1 -> GreaterThan1/1
  Constant7/1 -> Vector Concatenate/4
  raptor_adjustment5/1 -> GreaterThan1/2
  for 0.01% inc/1 -> raptor_override21/1
  Add2/1 -> Divide/2
  Conv. to Hz/1 -> raptor_override20/1
  GreaterThan1/1 -> raptor_fault_def/1
  Constant4/1 -> Switch1/3
  Constant1/1 -> Add/1
  raptor_fault_status/1 -> raptor_measurement21/1, Logical Operator3/1
  raptor_fault_status1/1 -> raptor_measurement22/1, Logical Operator3/2
  raptor_fault_status2/1 -> raptor_measurement23/1, Logical Operator3/3
  raptor_fault_status3/1 -> raptor_measurement24/1, Logical Operator3/4
  raptor_fault_status4/1 -> raptor_measurement25/1, Logical Operator3/5
  raptor_fault_status5/1 -> Logical Operator3/6, raptor_measurement26/1
  Logical Operator3/1 -> raptor_override14/1
  raptor_analog_in/1 -> POT1/1
  raptor_analog_in1/1 -> POT2/1
  raptor_override3/1 -> raptor_measurement4/1, Calculate Torque/2(RPM)
  raptor_override2/1 -> raptor_measurement12/1, raptor_digital_out/1
  Switch/1 -> Calculate Torque/1(APP%), raptor_measurement5/1
  raptor_override8/1 -> Mux/1, raptor_measurement6/1
  raptor_override9/1 -> Mux/2, raptor_measurement7/1
  raptor_override11/1 -> raptor_measurement10/1, Logical Operator1/2
  Compare To Constant1/1 -> raptor_measurement11/1, Logical Operator/2
  Calculate Torque/1(Actual Torque) -> raptor_override16/1
  Abs/1 -> raptor_override3/1
  raptor_override12/1 -> raptor_measurement13/1, Product3/1
  raptor_override13/1 -> I: R (kOhm) O: T (C)/1, raptor_measurement14/1
  raptor_override14/1 -> raptor_measurement17/1, Logical Operator7/1
  raptor_override15/1 -> Switch/1
  raptor_analog_in5/1 -> raptor_override7/1
  raptor_override7/1 -> Sum/1, raptor_measurement15/1
  Constant2/1 -> Sum/2, Divide1/2
  Sum/1 -> Divide1/1
  Constant3/1 -> Product1/2
  Divide1/1 -> Product1/1
  Product1/1 -> GLV Used Ah/1(In1), raptor_measurement16/1
  raptor_override16/1 -> Command Troque/1(Requested Torque)
  raptor_override17/1 -> Switch/3
  Conv. to Hz1/1 -> raptor_override19/1
  Q (L/H) vs. F (Hz)/1 -> Conv. to Hz1/1
  raptor_override19/1 -> Difference1/1, raptor_measurement19/1, Less Than2/1
  Compare To Constant2/1 -> raptor_override2/1
  raptor_override18/1 -> I: Temp. () O: Power (W)/1, Difference/1, Switch2/1, raptor_measurement27/1
  Delay/1 -> Switch2/2
  25C default/1 -> Switch2/3
  Switch2/1 -> GreaterThan4/1
  Enable switch/1 -> Delay/1
  raptor_override20/1 -> raptor_measurement18/1, Q (L/H) vs. F (Hz)/1
  Switch3/1 -> for 0.01% inc1/1
  Constant6/1 -> Switch3/3
  raptor_override10/1 -> Switch3/2, Switch1/2, Command Troque/2(Inverter Enable), Triggered Single Pulse/1(Trigger), raptor_measurement9/1, Switch/2
  raptor_adjustment8/1 -> Switch3/1
  raptor_adjustment1/1 -> for 0.01% inc2/1
  for 0.01% inc1/1 -> raptor_pwm_out1/1
  for 0.01% inc2/1 -> raptor_pwm_out1/2
  for 0.01% inc3/1 -> raptor_pwm_out/2
  I: 0-80W O: DC/1 -> Switch1/1
  raptor_override21/1 -> raptor_measurement28/1, raptor_pwm_out/1
  raptor_analog_in6/1 -> raptor_override22/1
  raptor_override22/1 -> Compare To Constant3/1
  Compare To Constant3/1 -> Logical Operator5/1, raptor_measurement29/1
  Logical Operator4/1 -> Logical Operator5/2
  Logical Operator5/1 -> raptor_override24/1, Logical Operator6/1
  Logical Operator6/1 -> raptor_measurement30/1, raptor_override23/1
  raptor_override23/1 -> raptor_digital_out2/1
  raptor_override24/1 -> raptor_measurement31/1, raptor_digital_out1/1
  Logical Operator7/1 -> Logical Operator1/5
  Mod/1 -> GLV Used Ah/Trigger
  Constant8/1 -> Mod/2
  raptor_time/1 -> Mod/1
